simulink model "mTruckPlatoon"  (R2018b)
settings: Solver=VariableStepAuto  StartTime=0.0  StopTime=simTime  RelTol=1e-3
PreLoadFcn:
  | load 'tableStructure.mat'
InitFcn:
  | clear actorCount;
  | clear plotStats;
  | modelParams
StopFcn:
  | delete 'roadInfo.mat'
values from neighbouring files (symbols this model uses):
  initYPos = 0    [modelParams.m]
  numTrucks = 0    [modelParams.m]
  sensorRange = 600    [modelParams.m]
  truckIdBase = 0    [modelParams.m]
  truckVelocity = 0    [modelParams.m]
  truckXPosition = 0    [modelParams.m]
libraries: smartTruckLib x6, dataTableBlockslib x2
settings Model: Creator=surongal  LastModifiedBy=surongal
settings DataIOCC: SaveTime=off  ReturnWorkspaceOutputs=on
settings DebuggingCC: InheritedTsInSrcMsg=none
settings SFSimCC: SimUseLocalCustomCode=off
settings RTWCC: RTWUseLocalCustomCode=off

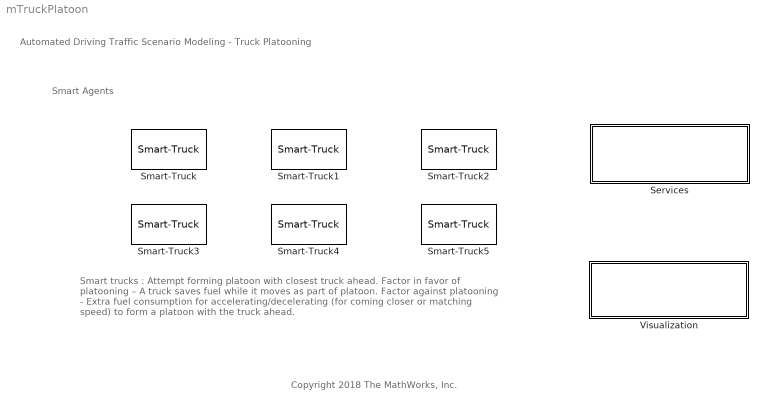
== system mTruckPlatoon ==
  note: Smart Agents
  note: Copyright 2018 The MathWorks, Inc.
  note: Smart trucks : Attempt forming platoon with closest truck ahead.
      | Factor in favor of platooning – A truck saves fuel while it moves as part of platoon.
      | Factor against platooning - Extra fuel consumption for accelerating/decelerating (for coming closer or matching speed) to form a platoon with the truck ahead.
  note: Automated Driving Traffic Scenario Modeling - Truck Platooning
  Services : Subsystem
      mask Display: disp('Services');
  Smart-Truck : smartTruckLib/Smart-Truck  initXPos=100  destXPos=4800  initXVel=10  maxAcceleration=3  maxDeceleration=-6  maxVelocity=20  truckId=1
  Smart-Truck1 : smartTruckLib/Smart-Truck  initXPos=200  destXPos=2500  initXVel=12  maxAcceleration=3  maxDeceleration=-6  maxVelocity=20  truckId=2
  Smart-Truck2 : smartTruckLib/Smart-Truck  initXPos=550  destXPos=1600  initXVel=15  maxAcceleration=3  maxDeceleration=-6  maxVelocity=25  truckId=3
  Smart-Truck3 : smartTruckLib/Smart-Truck  initXPos=450  destXPos=3500  initXVel=15  maxAcceleration=3  maxDeceleration=-6  maxVelocity=30  truckId=4
  Smart-Truck4 : smartTruckLib/Smart-Truck  initXPos=350  destXPos=1250  initXVel=10  maxAcceleration=3  maxDeceleration=-6  maxVelocity=20  truckId=5
  Smart-Truck5 : smartTruckLib/Smart-Truck  initXPos=600  destXPos=3500  initXVel=12  maxAcceleration=3  maxDeceleration=-6  maxVelocity=20  truckId=6
  Visualization : Subsystem
      mask Display: disp('Visualization');

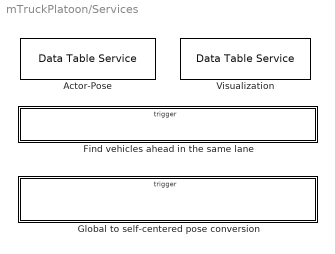
== system mTruckPlatoon/Services ==
  Actor-Pose : dataTableBlockslib/Data Table Service  tableName=Actor  tableSize=30  tableFormat=Vehicle  tableQueries={{PlatooningQueries.VehiclesAhead,'findVehiclesAhead'}}  mask(DataTableService){}
      mask Display: disp('Actor Pose Information')
  Find vehicles ahead in the same lane : Subsystem  TreatAsAtomicUnit=on
  Global to self-centered pose conversion : Subsystem  TreatAsAtomicUnit=on
  "Visualization " : dataTableBlockslib/Data Table Service  tableName=Visualization  tableSize=30  tableFormat=PlatoonStatistics  tableQueries={}  mask(DataTableService){}
      mask Display: disp('Platoon Information')

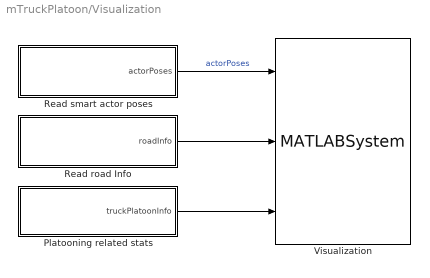
== system mTruckPlatoon/Visualization ==
  Platooning related stats : MATLAB Function  TreatAsAtomicUnit=on
  Read road Info : MATLAB Function  TreatAsAtomicUnit=on
  Read smart actor poses : MATLAB Function  TreatAsAtomicUnit=on
  Visualization : MATLABSystem  StopFcn=""  System=visualizer
      mask Type: visualizer
      mask Display:
      | disp('Visualizer');
      | port_label('input',1,'Actors');
      | port_label('input',2,'Roads');
      | port_label('input',3,'Statistics');
  wires:
  Read road Info/1(roadInfo) -> Visualization/2
  Platooning related stats/1(truckPlatoonInfo) -> Visualization/3
  Read smart actor poses/1(actorPoses) -> Visualization/1  "actorPoses"

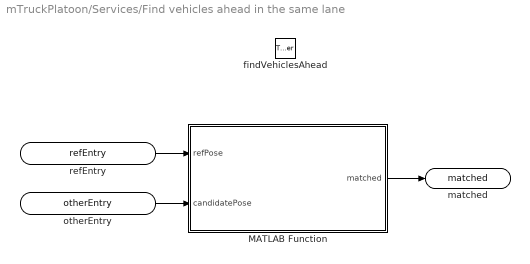
== system mTruckPlatoon/Services/Find vehicles ahead in the same lane ==
  findVehiclesAhead : TriggerPort  TriggerType=function-call  IsSimulinkFunction=on  FunctionName=findVehiclesAhead  FunctionVisibility=scoped  VariantControl=(inherit)
  MATLAB Function : MATLAB Function  TreatAsAtomicUnit=on
  refEntry : ArgIn  OutDataTypeStr=Bus: Vehicle  ArgumentName=refEntry
  otherEntry : ArgIn  Port=2  OutDataTypeStr=Bus: Vehicle  ArgumentName=otherEntry
  matched : ArgOut  DisableCoverage=on  OutDataTypeStr=boolean  ArgumentName=matched
  wires:
  MATLAB Function/1(matched) -> matched/1
  refEntry/1 -> MATLAB Function/1(refPose)
  otherEntry/1 -> MATLAB Function/2(candidatePose)

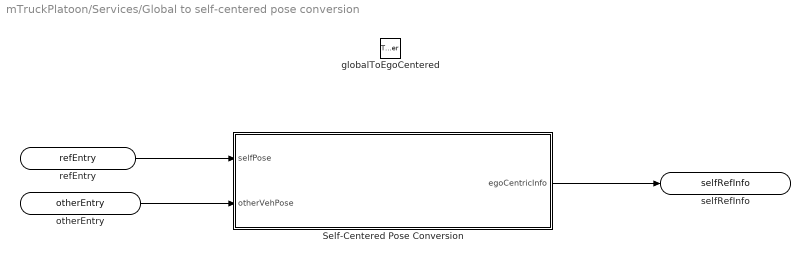
== system mTruckPlatoon/Services/Global to self-centered pose conversion ==
  globalToEgoCentered : TriggerPort  TriggerType=function-call  IsSimulinkFunction=on  FunctionName=globalToEgoCentered  VariantControl=(inherit)
  Self-Centered Pose Conversion : MATLAB Function  TreatAsAtomicUnit=on
  refEntry : ArgIn  DisableCoverage=on  OutDataTypeStr=Bus: Vehicle  ArgumentName=refEntry
  otherEntry : ArgIn  Port=2  OutDataTypeStr=Bus: Vehicle  ArgumentName=otherEntry
  selfRefInfo : ArgOut  DisableCoverage=on  OutDataTypeStr=Bus: Vehicle  ArgumentName=selfRefInfo
  wires:
  refEntry/1 -> Self-Centered Pose Conversion/1(selfPose)
  otherEntry/1 -> Self-Centered Pose Conversion/2(otherVehPose)
  Self-Centered Pose Conversion/1(egoCentricInfo) -> selfRefInfo/1

== matlab function mTruckPlatoon/Services/Find vehicles ahead in the same lane/MATLAB Function ==
  data: refPose input; matched output; candidatePose input; sensorRange parameter; initYPos parameter
function matched = findVehiclesAheadSameLane(refPose, candidatePose, sensorRange, initYPos)
% For any vehicle, get the vehicles ahead. Query is assumed
% to called for a vehicle moving in +ve X direction
% refPose - Query-Calling vehicle
% candidatePose - Actor to be processed as candidate for matching the query criteria.

if ((candidatePose.Position(1) - refPose.Position(1)) > 0 && ...
        (candidatePose.Position(1) - refPose.Position(1) < sensorRange) && candidatePose.Position(2) == initYPos)
    matched = true;
else
    matched = false;
end

== matlab function mTruckPlatoon/Visualization/Read road Info ==
  data: roadInfo output; roadInfoFileNameU parameter
function roadInfo = getRoadBoundaries(roadInfoFileNameU)
% Read the road boundaries information

roadData = load(char(roadInfoFileNameU));
roadInfo = roadData.RoadBoundaries;

== matlab function mTruckPlatoon/Visualization/Read smart actor poses ==
  data: truckIdBase parameter; numTrucks parameter; actorPoses output Bus: Vehicle; truckXPosition parameter; truckVelocity parameter; initYPos parameter
function actorPoses = getTruckPose(truckIdBase, numTrucks, truckXPosition, ...
                                      truckVelocity, initYPos)
% Read poses of trucks (from data table)

actorStruct = struct('ActorID', 0, 'Position', [0 0 0], ...
    'Velocity', [0 0 0], 'Roll', 0, 'Pitch', 0, 'Yaw', 0, ...
    'AngularVelocity', [0 0 0]);
% Create an actor structure array for all required actors
truckPoses = repmat(actorStruct, [numTrucks, 1]);

for i = 1 : numTrucks % For all the trucks.
    % Getting the key corresponding to the actorId from the data table.
    % As Actor-Id is the first field in the actor-pose info, field-index is
    % passed as '1'.
    key = getActorTableEntryKey(uint32(1), (truckIdBase + i));
    if key ~= -1
        % Retrieve the actor details based on key
        truckPoses(i) = getActorTableEntry(key);
    else
        % Fill the inital pose info as filled in mask paramters of trucks.
        truckPoses(i).ActorID = truckIdBase + i;
        truckPoses(i).Position(1) = truckXPosition(i);
        truckPoses(i).Position(2) = initYPos;
        truckPoses(i).Velocity(1) = truckVelocity(i);
    end
end
actorPoses = truckPoses;

== matlab function mTruckPlatoon/Visualization/Platooning related stats ==
  data: truckPlatoonInfo output Bus: PlatoonStatistics; truckIdBase parameter; numTrucks parameter
function truckPlatoonInfo = getPlatoonStats(truckIdBase, numTrucks)
% Get platooning related stats for sending to visulizer.

actorStruct = struct('ActorID', 0, 'VehicleAheadID', 0, 'PlatoonStatus', 0, 'FuelSavings', 0);
truckPlatoonInfo = repmat(actorStruct, [numTrucks 1]);
for i = 1 : numTrucks % For all the trucks.
    % Getting the key corresponding to the actorId from the data table.
     % As Actor-Id is the first field in the actor-pose info, field-index is
    % passed as '1'.
    key = getVisualizationTableEntryKey(uint32(1), (truckIdBase + i));
    if key ~= -1 
        % Retrieve the actor details based on key
        truckPlatoonInfo(i) = getVisualizationTableEntry(key);
    else % No valid entry.
        truckPlatoonInfo(i).ActorID = (truckIdBase + i);
        truckPlatoonInfo(i).VehicleAheadID = 0;
        truckPlatoonInfo(i).PlatoonStatus = 0;
        truckPlatoonInfo(i).FuelSavings = 0;
        setVisualizationTableEntry(truckPlatoonInfo(i).ActorID,truckPlatoonInfo(i));
    end
end

== matlab function mTruckPlatoon/Services/Global to self-centered pose conversion/Self-Centered Pose Conversion ==
  data: selfPose input; otherVehPose input Bus: Vehicle; egoCentricInfo output Bus: Vehicle
function egoCentricInfo = globalToEgoCenteredConversion(selfPose, otherVehPose)
% Convert global-coordinate pose of another vehicle to self-centered pose.

egoCentricInfo.ActorID = otherVehPose.ActorID;
egoCentricInfo.Position = otherVehPose.Position - selfPose.Position;
egoCentricInfo.Velocity = otherVehPose.Velocity - selfPose.Velocity;
egoCentricInfo.Roll = otherVehPose.Roll - selfPose.Roll;
egoCentricInfo.Pitch = otherVehPose.Pitch - selfPose.Pitch;
egoCentricInfo.Yaw = otherVehPose.Yaw - selfPose.Yaw;
egoCentricInfo.AngularVelocity = otherVehPose.AngularVelocity - selfPose.AngularVelocity;
